simulink model "Ssim_OF"  (Simulink 10.2)
settings: Solver=VariableStepAuto  StartTime=0.0  StopTime=10  FixedStep=0.001  RelTol=1e-3  EnableMultiTasking=on
libraries: simulink x1
settings Model: Creator=hp  LastModifiedBy=11634
settings SolverCC: AlgebraicLoopSolver=LineSearch
settings DataIOCC: LimitDataPoints=on  SignalLoggingName=sigsOut
settings OptimizationCC: ExpressionDepthLimit=2147483647  InitFltsAndDblsToZero=on
settings DebuggingCC: SaveWithParameterizedLinksMsg=none  SignalResolutionControl=TryResolveAllWithWarning  MultiTaskDSMMsg=warning  MultiTaskCondExecSysMsg=none  StateNameClashWarn=warning
settings HardwareCC: TargetUnknown=on
settings GRTTargetCC: TargetFcnLib=ansi_tfl_tmw.mat

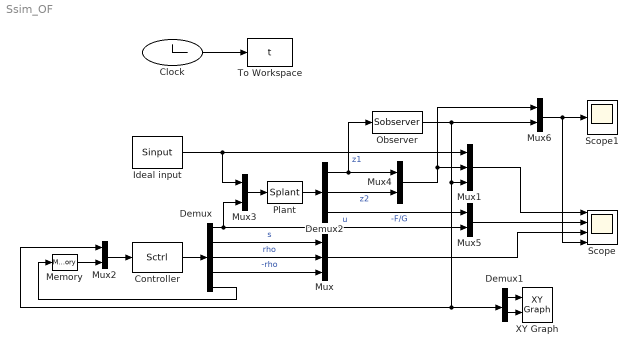
== system Ssim_OF ==
  Clock : Clock
  Controller : S-Function  FunctionName=Sctrl  SFunctionDeploymentMode=off  EnableBusSupport=off
  Demux : Demux  Outputs=5
  Demux1 : Demux  Outputs=2
  Demux2 : Demux  Outputs=3
  Ideal input : S-Function  FunctionName=Sinput  SFunctionDeploymentMode=off  EnableBusSupport=off
  Memory : Memory
  Mux : Mux  Inputs=3
  Mux1 : Mux  Inputs=3
  Mux{2..6} (5 alike) : Mux  Inputs=2
  Observer : S-Function  FunctionName=Sobserver  SFunctionDeploymentMode=off  EnableBusSupport=off
  Plant : S-Function  FunctionName=Splant  SFunctionDeploymentMode=off  EnableBusSupport=off
  Scope : Scope  NumInputPorts=4
  Scope1 : Scope
  To Workspace : ToWorkspace  VariableName=t  SampleTime=-1
  XY Graph : simulink/Sinks/XY Graph  xmin=-1  xmax=1.5  ymin=-1  ymax=1.5  st=-1
  wires:
  Demux/1 -> Mux5/2, Mux3/2  "u"
  Observer/1 -> Mux1/3, Demux1/1, Mux2/1, Mux6/2
  Clock/1 -> To Workspace/1
  Ideal input/1 -> Mux3/1, Mux1/1
  Mux1/1 -> Scope/1
  Controller/1 -> Demux/1
  Mux/1 -> Scope/3
  Demux1/1 -> XY Graph/1
  Demux1/2 -> XY Graph/2
  Demux/2 -> Mux/1  "s"
  Demux/3 -> Mux/2  "rho"
  Demux/4 -> Mux/3  "-rho"
  Demux2/1 -> Observer/1, Mux4/1  "z1"
  Plant/1 -> Demux2/1
  Demux2/3 -> Mux5/1  "-F/G"
  Mux5/1 -> Scope/2
  Demux2/2 -> Mux4/2  "z2"
  Mux4/1 -> Mux6/1, Mux1/2
  Mux6/1 -> Scope/4, Scope1/1
  Mux3/1 -> Plant/1
  Mux2/1 -> Controller/1
  Memory/1 -> Mux2/2
  Demux/5 -> Memory/1
